simulink model "aero_dap3dof"  (R2018a)
settings: Solver=ode45  StartTime=0  StopTime=25  FixedStep=clockt/4  RelTol=1e-3  AbsTol=1e-6
PreLoadFcn:
  | aero_dap3dofdata
undefined symbols (not defined in the file): alph1, alphs1, DB, delt, Force, I, L_arm
libraries: aero_libdap x1, aero_librcs x1
CloseFcn:
  | h=findobj('type','figure','Name','aero_dap3dof');if ~isempty(h);close(h);end
Description:
  | Apollo Lunar Module Digital Autopilot
  | 
  | This model was featured in "Fly Me to the Moon - Then and Now", the story of the digital
  | autopilot in the Lunar Module from the Summer 1999 issue of "MATLAB(R) News & Notes".
  | Double click on the link in the model to view the article online over the Internet.
settings Model: RequirementInfo=9  ExtModeTrigMode=oneshot  ExtModeArmWhenConnect=off  ExtModeAutoUpdateStatusClock=off  Creator=The MathWorks, Inc.  LastModifiedBy=The MathWorks, Inc.
settings SolverCC: AutoScaleAbsTol=off
settings DataIOCC: SaveFormat=Array  SignalLoggingName=logsOut
settings OptimizationCC: BlockReduction=off  ExpressionDepthLimit=2147483647  InitFltsAndDblsToZero=on  LifeSpan=inf
settings DebuggingCC: SaveWithParameterizedLinksMsg=none  SignalResolutionControl=TryResolveAllWithWarning  MultiTaskDSMMsg=warning  MultiTaskCondExecSysMsg=none  SigSpecEnsureSampleTimeMsg=none  FcnCallInpInsideContextMsg=warning  StateNameClashWarn=warning  SFUnexpectedBacktrackingDiag=warning  SFNoUnconditionalDefaultTransitionDiag=warning  SFExecutionAtInitializationDiag=none
settings HardwareCC: ProdBitPerPointer=32  ProdBitPerSizeT=32  ProdBitPerPtrDiffT=32  ProdLargestAtomicFloat=None  ProdIntDivRoundTo=Undefined  ProdEndianess=Unspecified  ProdWordSize=32  ProdHWDeviceType=Specified
settings ModelReferenceCC: PropagateSignalLabelsOutOfModel=off
settings SFSimCC: SimParseCustomCode=off
settings RTWCC: TemplateMakefile=grt_vc.tmf
settings CodeAppCC: StateflowObjectComments=on
settings GRTTargetCC: TargetFcnLib=ansi_tfl_tmw.mat  TargetLangStandard=C89/C90 (ANSI)  GeneratePreprocessorConditionals=Disable all  CombineOutputUpdateFcns=off  GRTInterface=on
settings ConfigComp: CovMetricSettings=d  CovHtmlReporting=on  CovSaveCumulativeToWorkspaceVar=on  CovSaveSingleToWorkspaceVar=on  CovExternalEMLEnable=off

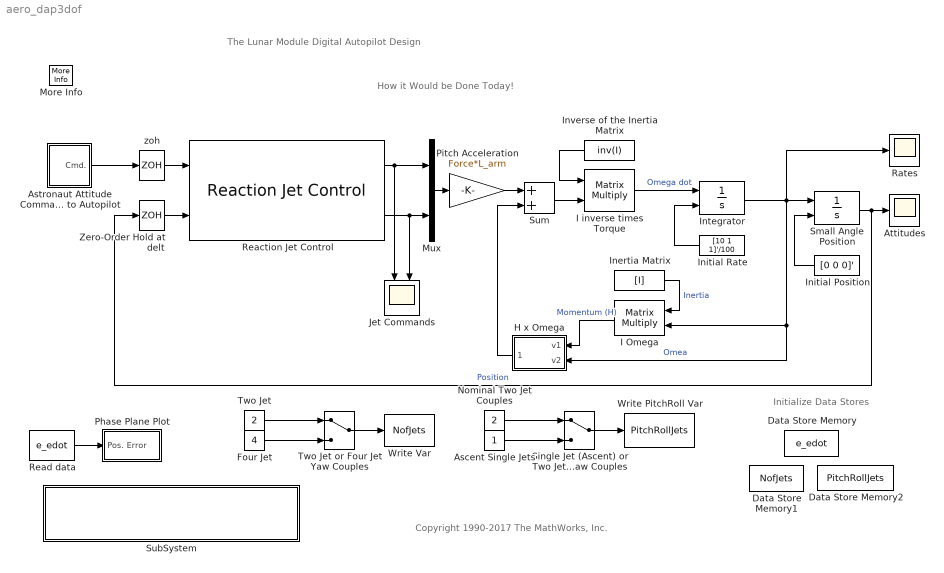
== system aero_dap3dof ==
  note: The Lunar Module Digital Autopilot Design
  note: How it Would be Done Today!
  note: Initialize Data Stores
  note: Copyright 1990-2017 The MathWorks, Inc.
  Ascent Single Jets : Constant
  Astronaut Attitude Command to Autopilot : Subsystem
  Attitudes : Scope
  Data Store Memory : DataStoreMemory  DataStoreName=e_edot  InitialValue=[0 0]  ShowAdditionalParam=off
  Data Store Memory1 : DataStoreMemory  DataStoreName=NofJets  InitialValue=2  ShowAdditionalParam=off
  Data Store Memory2 : DataStoreMemory  DataStoreName=PitchRollJets  InitialValue=2  ShowAdditionalParam=off
  Four Jet : Constant  Value=4
  H x Omega : Subsystem  mask(Vector Cross Product){}
      mask help: This block computes the vector cross product of the first input with the second input. The output is then z= v1 x v2.
  I Omega : Product  Multiplication=Matrix(*)  SaturateOnIntegerOverflow=on  RndMeth=Zero  InputSameDT=on  OutDataTypeStr=Inherit: Same as first input
  I inverse times Torque : Product  Multiplication=Matrix(*)  SaturateOnIntegerOverflow=on  RndMeth=Zero  InputSameDT=on  OutDataTypeStr=Inherit: Same as first input
  Inertia Matrix : Constant  Value=[I]  VectorParams1D=off
  Initial Position : Constant  Value=[0 0 0]'  VectorParams1D=off
  Initial Rate : Constant  Value=[10 1 1]'/100  VectorParams1D=off
  Integrator : Integrator  InitialConditionSource=external
  Inverse of the Inertia Matrix : Constant  Value=inv(I)  VectorParams1D=off
  Jet Commands : Scope  NumInputPorts=2
  More Info : aero_libdap/More Info  SystemSampleTime=-1
      settings: SourceProductName=Simulink  SourceProductBaseCode=SL
  Mux : Mux  Inputs=2
  Nominal Two Jet Couples : Constant  Value=2
  Phase Plane Plot : Subsystem
  Pitch Acceleration : Gain  Gain=Force*L_arm  SaturateOnIntegerOverflow=on  OutDataTypeStr=Inherit: Same as input  ParamDataTypeStr=Inherit: Same as input
  Rates : Scope
  Reaction Jet Control : aero_librcs/Reaction Jet Control
      settings: SourceProductName=Simulink  SourceProductBaseCode=SL
  Read data : DataStoreRead  DataStoreName=e_edot  SampleTime=delt
  Single Jet (Ascent) or Two Jet Yaw Couples : ManualSwitch
  Small Angle Position : Integrator  InitialConditionSource=external
  SubSystem : Subsystem
      mask init:
      | dispstr = sprintf('Read the "News & Notes" article\nabout this model over the web.\n(Double-Click Here)');
      settings: OpenFcn=web https://www.mathworks.com/company/newsletters/articles/fly-me-to-the-moon-then-and-now.html
      mask Display: disp(dispstr)
  Sum : Sum  SaturateOnIntegerOverflow=on  InputSameDT=on  OutDataTypeStr=Inherit: Same as first input
  Two Jet : Constant  Value=2
  Two Jet or Four Jet Yaw Couples : ManualSwitch
  Write PitchRoll Var : DataStoreWrite  DataStoreName=PitchRollJets
  Write Var : DataStoreWrite  DataStoreName=NofJets
  Zero-Order Hold at delt : ZeroOrderHold  SampleTime=delt
  zoh : ZeroOrderHold  SampleTime=delt
  wires:
  Inverse of the Inertia Matrix/1 -> I inverse times Torque/1
  I inverse times Torque/1 -> Integrator/1  "Omega dot"
  Inertia Matrix/1 -> I Omega/1  "Inertia"
  Initial Rate/1 -> Integrator/2
  Initial Position/1 -> Small Angle Position/2
  Integrator/1 -> Small Angle Position/1, Rates/1, H x Omega/2(v2), I Omega/2  "Omea"
  Small Angle Position/1 -> Attitudes/1, Zero-Order Hold at delt/1  "Position"
  Sum/1 -> I inverse times Torque/2
  I Omega/1 -> H x Omega/1(v1)  "Momentum (H)"
  H x Omega/1(v1 x v2) -> Sum/2
  Astronaut Attitude Command to Autopilot/1(Cmd.) -> zoh/1
  Pitch Acceleration/1 -> Sum/1
  Mux/1 -> Pitch Acceleration/1
  Reaction Jet Control/1 -> Mux/1, Jet Commands/1
  Reaction Jet Control/2 -> Mux/2, Jet Commands/2
  zoh/1 -> Reaction Jet Control/1
  Zero-Order Hold at delt/1 -> Reaction Jet Control/2
  Ascent Single Jets/1 -> Single Jet (Ascent) or Two Jet Yaw Couples/2
  Nominal Two Jet Couples/1 -> Single Jet (Ascent) or Two Jet Yaw Couples/1
  Single Jet (Ascent) or Two Jet Yaw Couples/1 -> Write PitchRoll Var/1
  Four Jet/1 -> Two Jet or Four Jet Yaw Couples/2
  Two Jet/1 -> Two Jet or Four Jet Yaw Couples/1
  Two Jet or Four Jet Yaw Couples/1 -> Write Var/1
  Read data/1 -> Phase Plane Plot/1(Pos. Error)

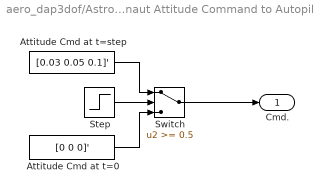
== system aero_dap3dof/Astronaut Attitude Command to Autopilot ==
  Attitude Cmd at t=0 : Constant  Value=[0 0 0]'  VectorParams1D=off
  Attitude Cmd at t=step : Constant  Value=[0.03 0.05 0.1]'  VectorParams1D=off
  Step : Step  Time=0.25  SampleTime=0
  Switch : Switch  Threshold=0.5  SaturateOnIntegerOverflow=on  InputSameDT=on
  Cmd. : Outport
  wires:
  Step/1 -> Switch/2
  Attitude Cmd at t=step/1 -> Switch/1
  Attitude Cmd at t=0/1 -> Switch/3
  Switch/1 -> Cmd./1

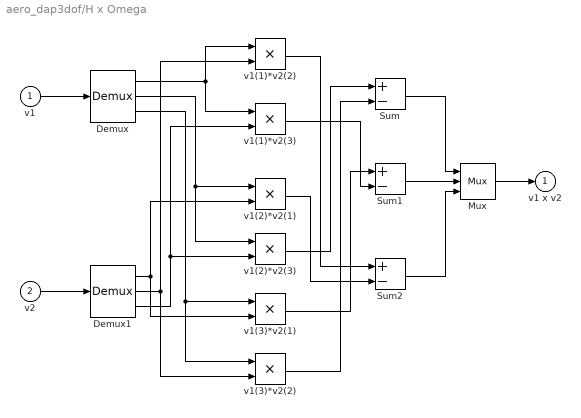
== system aero_dap3dof/H x Omega ==
  v1 : Inport
  v2 : Inport  Port=2
  Demux : Demux  Outputs=3
  Demux1 : Demux  Outputs=3
  Mux : Mux  Inputs=3
  Sum : Sum  Inputs=+-  SaturateOnIntegerOverflow=on  InputSameDT=on  OutDataTypeStr=Inherit: Same as first input
  Sum1 : Sum  Inputs=+-  SaturateOnIntegerOverflow=on  InputSameDT=on  OutDataTypeStr=Inherit: Same as first input
  Sum2 : Sum  Inputs=+-  SaturateOnIntegerOverflow=on  InputSameDT=on  OutDataTypeStr=Inherit: Same as first input
  v1(1)*v2(2) : Product  SaturateOnIntegerOverflow=on  RndMeth=Zero  InputSameDT=on  OutDataTypeStr=Inherit: Same as first input
  v1(1)*v2(3) : Product  SaturateOnIntegerOverflow=on  RndMeth=Zero  InputSameDT=on  OutDataTypeStr=Inherit: Same as first input
  v1(2)*v2(1) : Product  SaturateOnIntegerOverflow=on  RndMeth=Zero  InputSameDT=on  OutDataTypeStr=Inherit: Same as first input
  v1(2)*v2(3) : Product  SaturateOnIntegerOverflow=on  RndMeth=Zero  InputSameDT=on  OutDataTypeStr=Inherit: Same as first input
  v1(3)*v2(1) : Product  SaturateOnIntegerOverflow=on  RndMeth=Zero  InputSameDT=on  OutDataTypeStr=Inherit: Same as first input
  v1(3)*v2(2) : Product  SaturateOnIntegerOverflow=on  RndMeth=Zero  InputSameDT=on  OutDataTypeStr=Inherit: Same as first input
  v1 x v2 : Outport  InitialOutput=0
  wires:
  v1/1 -> Demux/1
  Demux/3 -> v1(3)*v2(1)/1, v1(3)*v2(2)/1
  v2/1 -> Demux1/1
  Demux1/1 -> v1(2)*v2(1)/2, v1(3)*v2(1)/2
  Demux1/2 -> v1(3)*v2(2)/2, v1(1)*v2(2)/2
  Demux1/3 -> v1(2)*v2(3)/2, v1(1)*v2(3)/2
  Demux/1 -> v1(1)*v2(2)/1, v1(1)*v2(3)/1
  Demux/2 -> v1(2)*v2(1)/1, v1(2)*v2(3)/1
  Mux/1 -> v1 x v2/1
  Sum/1 -> Mux/1
  Sum1/1 -> Mux/2
  Sum2/1 -> Mux/3
  v1(2)*v2(3)/1 -> Sum/1
  v1(3)*v2(2)/1 -> Sum/2
  v1(3)*v2(1)/1 -> Sum1/1
  v1(1)*v2(3)/1 -> Sum1/2
  v1(1)*v2(2)/1 -> Sum2/1
  v1(2)*v2(1)/1 -> Sum2/2

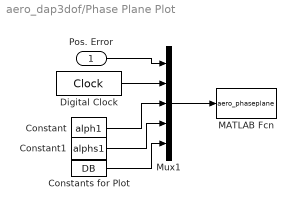
== system aero_dap3dof/Phase Plane Plot ==
  Pos. Error : Inport
  Constant : Constant  Value=alph1
  Constant1 : Constant  Value=alphs1
  Constants for Plot : Constant  Value=DB
  Digital Clock : DigitalClock  SampleTime=delt
  MATLAB Fcn : MATLABFcn  MATLABFcn=aero_phaseplane  OutputDimensions=0
  Mux1 : Mux  Inputs=5
  wires:
  Mux1/1 -> MATLAB Fcn/1
  Pos. Error/1 -> Mux1/1
  Digital Clock/1 -> Mux1/2
  Constants for Plot/1 -> Mux1/5
  Constant/1 -> Mux1/3
  Constant1/1 -> Mux1/4

== system aero_dap3dof/SubSystem ==
